simulink model "w3_warplab_agc"  (Simulink 7.7)
settings: Solver=ode45  StartTime=0.0  StopTime=1e4  RelTol=1e-3
PostLoadFcn:
  | w3_warplab_agc_init
InitFcn:
  | w3_warplab_agc_init
StartFcn:
  | w3_warplab_agc_init
undefined symbols (not defined in the file): gcbh, PHY_CONFIG_PKT_DET_CORR_THRESH, PHY_CONFIG_PKT_DET_ENERGY_THRESH, PHY_CONFIG_PKT_DET_MIN_DURR, xlBlockLoadCallback, xlGetNormalizedPeriod
libraries: xbsIndex_r4 x1039, xbsEDKLib_r4 x1, simulink x1
(part 2 of 7)

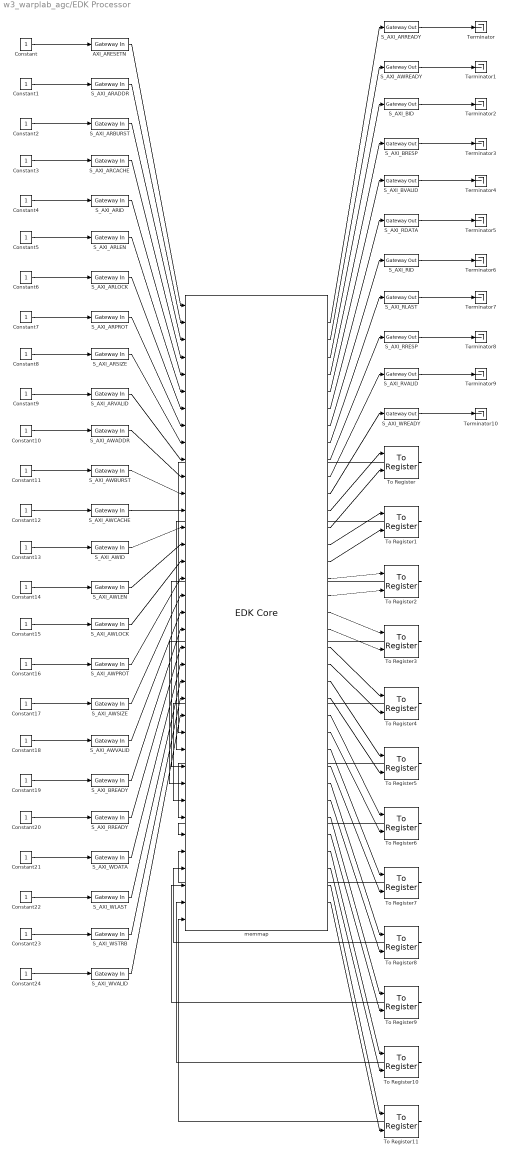
== system w3_warplab_agc/EDK Processor ==
  AXI_ARESETN : xbsIndex_r4/Gateway In  gui_display_data_type=Fixed-point  arith_type=Boolean  n_bits=16  bin_pt=14  preci_type=Single  exp_width=8  frac_width=24  quantization="Round  (unbiased: +/- Inf)"  overflow=Saturate  period=xlGetNormalizedPeriod()  dbl_ovrd=off  timing_constraint=None  locs_specified=off  LOCs={}  UseAsADC=off  ADCChannel='1'  inherit_from_input=off  hdl_port=on  block_type=gatewayin
  Constant{,1..24} (25 alike) : Constant
  S_AXI_ARADDR : xbsIndex_r4/Gateway In  gui_display_data_type=Fixed-point  arith_type=Unsigned  n_bits=32  bin_pt=0  preci_type=Single  exp_width=8  frac_width=24  quantization="Round  (unbiased: +/- Inf)"  overflow=Saturate  period=xlGetNormalizedPeriod()  dbl_ovrd=off  timing_constraint=None  locs_specified=off  LOCs={}  UseAsADC=off  ADCChannel='1'  inherit_from_input=off  hdl_port=on  block_type=gatewayin
  S_AXI_ARBURST : xbsIndex_r4/Gateway In  gui_display_data_type=Fixed-point  arith_type=Unsigned  n_bits=2  bin_pt=0  preci_type=Single  exp_width=8  frac_width=24  quantization="Round  (unbiased: +/- Inf)"  overflow=Saturate  period=xlGetNormalizedPeriod()  dbl_ovrd=off  timing_constraint=None  locs_specified=off  LOCs={}  UseAsADC=off  ADCChannel='1'  inherit_from_input=off  hdl_port=on  block_type=gatewayin
  S_AXI_ARCACHE : xbsIndex_r4/Gateway In  gui_display_data_type=Fixed-point  arith_type=Unsigned  n_bits=4  bin_pt=0  preci_type=Single  exp_width=8  frac_width=24  quantization="Round  (unbiased: +/- Inf)"  overflow=Saturate  period=xlGetNormalizedPeriod()  dbl_ovrd=off  timing_constraint=None  locs_specified=off  LOCs={}  UseAsADC=off  ADCChannel='1'  inherit_from_input=off  hdl_port=on  block_type=gatewayin
  S_AXI_ARID : xbsIndex_r4/Gateway In  gui_display_data_type=Fixed-point  arith_type=Unsigned  n_bits=8  bin_pt=0  preci_type=Single  exp_width=8  frac_width=24  quantization="Round  (unbiased: +/- Inf)"  overflow=Saturate  period=xlGetNormalizedPeriod()  dbl_ovrd=off  timing_constraint=None  locs_specified=off  LOCs={}  UseAsADC=off  ADCChannel='1'  inherit_from_input=off  hdl_port=on  block_type=gatewayin
  S_AXI_ARLEN : xbsIndex_r4/Gateway In  gui_display_data_type=Fixed-point  arith_type=Unsigned  n_bits=8  bin_pt=0  preci_type=Single  exp_width=8  frac_width=24  quantization="Round  (unbiased: +/- Inf)"  overflow=Saturate  period=xlGetNormalizedPeriod()  dbl_ovrd=off  timing_constraint=None  locs_specified=off  LOCs={}  UseAsADC=off  ADCChannel='1'  inherit_from_input=off  hdl_port=on  block_type=gatewayin
  S_AXI_ARLOCK : xbsIndex_r4/Gateway In  gui_display_data_type=Fixed-point  arith_type=Unsigned  n_bits=2  bin_pt=0  preci_type=Single  exp_width=8  frac_width=24  quantization="Round  (unbiased: +/- Inf)"  overflow=Saturate  period=xlGetNormalizedPeriod()  dbl_ovrd=off  timing_constraint=None  locs_specified=off  LOCs={}  UseAsADC=off  ADCChannel='1'  inherit_from_input=off  hdl_port=on  block_type=gatewayin
  S_AXI_ARPROT : xbsIndex_r4/Gateway In  gui_display_data_type=Fixed-point  arith_type=Unsigned  n_bits=3  bin_pt=0  preci_type=Single  exp_width=8  frac_width=24  quantization="Round  (unbiased: +/- Inf)"  overflow=Saturate  period=xlGetNormalizedPeriod()  dbl_ovrd=off  timing_constraint=None  locs_specified=off  LOCs={}  UseAsADC=off  ADCChannel='1'  inherit_from_input=off  hdl_port=on  block_type=gatewayin
  S_AXI_ARREADY : xbsIndex_r4/Gateway Out  inherit_from_input=off  hdl_port=on  timing_constraint=None  locs_specified=off  LOCs={}  UseAsDAC=off  DACChannel='1'  block_type=gatewayout
  S_AXI_ARSIZE : xbsIndex_r4/Gateway In  gui_display_data_type=Fixed-point  arith_type=Unsigned  n_bits=3  bin_pt=0  preci_type=Single  exp_width=8  frac_width=24  quantization="Round  (unbiased: +/- Inf)"  overflow=Saturate  period=xlGetNormalizedPeriod()  dbl_ovrd=off  timing_constraint=None  locs_specified=off  LOCs={}  UseAsADC=off  ADCChannel='1'  inherit_from_input=off  hdl_port=on  block_type=gatewayin
  S_AXI_ARVALID : xbsIndex_r4/Gateway In  gui_display_data_type=Fixed-point  arith_type=Boolean  n_bits=16  bin_pt=14  preci_type=Single  exp_width=8  frac_width=24  quantization="Round  (unbiased: +/- Inf)"  overflow=Saturate  period=xlGetNormalizedPeriod()  dbl_ovrd=off  timing_constraint=None  locs_specified=off  LOCs={}  UseAsADC=off  ADCChannel='1'  inherit_from_input=off  hdl_port=on  block_type=gatewayin
  S_AXI_AWADDR : xbsIndex_r4/Gateway In  gui_display_data_type=Fixed-point  arith_type=Unsigned  n_bits=32  bin_pt=0  preci_type=Single  exp_width=8  frac_width=24  quantization="Round  (unbiased: +/- Inf)"  overflow=Saturate  period=xlGetNormalizedPeriod()  dbl_ovrd=off  timing_constraint=None  locs_specified=off  LOCs={}  UseAsADC=off  ADCChannel='1'  inherit_from_input=off  hdl_port=on  block_type=gatewayin
  S_AXI_AWBURST : xbsIndex_r4/Gateway In  gui_display_data_type=Fixed-point  arith_type=Unsigned  n_bits=2  bin_pt=0  preci_type=Single  exp_width=8  frac_width=24  quantization="Round  (unbiased: +/- Inf)"  overflow=Saturate  period=xlGetNormalizedPeriod()  dbl_ovrd=off  timing_constraint=None  locs_specified=off  LOCs={}  UseAsADC=off  ADCChannel='1'  inherit_from_input=off  hdl_port=on  block_type=gatewayin
  S_AXI_AWCACHE : xbsIndex_r4/Gateway In  gui_display_data_type=Fixed-point  arith_type=Unsigned  n_bits=4  bin_pt=0  preci_type=Single  exp_width=8  frac_width=24  quantization="Round  (unbiased: +/- Inf)"  overflow=Saturate  period=xlGetNormalizedPeriod()  dbl_ovrd=off  timing_constraint=None  locs_specified=off  LOCs={}  UseAsADC=off  ADCChannel='1'  inherit_from_input=off  hdl_port=on  block_type=gatewayin
  S_AXI_AWID : xbsIndex_r4/Gateway In  gui_display_data_type=Fixed-point  arith_type=Unsigned  n_bits=8  bin_pt=0  preci_type=Single  exp_width=8  frac_width=24  quantization="Round  (unbiased: +/- Inf)"  overflow=Saturate  period=xlGetNormalizedPeriod()  dbl_ovrd=off  timing_constraint=None  locs_specified=off  LOCs={}  UseAsADC=off  ADCChannel='1'  inherit_from_input=off  hdl_port=on  block_type=gatewayin
  S_AXI_AWLEN : xbsIndex_r4/Gateway In  gui_display_data_type=Fixed-point  arith_type=Unsigned  n_bits=8  bin_pt=0  preci_type=Single  exp_width=8  frac_width=24  quantization="Round  (unbiased: +/- Inf)"  overflow=Saturate  period=xlGetNormalizedPeriod()  dbl_ovrd=off  timing_constraint=None  locs_specified=off  LOCs={}  UseAsADC=off  ADCChannel='1'  inherit_from_input=off  hdl_port=on  block_type=gatewayin
  S_AXI_AWLOCK : xbsIndex_r4/Gateway In  gui_display_data_type=Fixed-point  arith_type=Unsigned  n_bits=2  bin_pt=0  preci_type=Single  exp_width=8  frac_width=24  quantization="Round  (unbiased: +/- Inf)"  overflow=Saturate  period=xlGetNormalizedPeriod()  dbl_ovrd=off  timing_constraint=None  locs_specified=off  LOCs={}  UseAsADC=off  ADCChannel='1'  inherit_from_input=off  hdl_port=on  block_type=gatewayin
  S_AXI_AWPROT : xbsIndex_r4/Gateway In  gui_display_data_type=Fixed-point  arith_type=Unsigned  n_bits=3  bin_pt=0  preci_type=Single  exp_width=8  frac_width=24  quantization="Round  (unbiased: +/- Inf)"  overflow=Saturate  period=xlGetNormalizedPeriod()  dbl_ovrd=off  timing_constraint=None  locs_specified=off  LOCs={}  UseAsADC=off  ADCChannel='1'  inherit_from_input=off  hdl_port=on  block_type=gatewayin
  S_AXI_AWREADY : xbsIndex_r4/Gateway Out  inherit_from_input=off  hdl_port=on  timing_constraint=None  locs_specified=off  LOCs={}  UseAsDAC=off  DACChannel='1'  block_type=gatewayout
  S_AXI_AWSIZE : xbsIndex_r4/Gateway In  gui_display_data_type=Fixed-point  arith_type=Unsigned  n_bits=3  bin_pt=0  preci_type=Single  exp_width=8  frac_width=24  quantization="Round  (unbiased: +/- Inf)"  overflow=Saturate  period=xlGetNormalizedPeriod()  dbl_ovrd=off  timing_constraint=None  locs_specified=off  LOCs={}  UseAsADC=off  ADCChannel='1'  inherit_from_input=off  hdl_port=on  block_type=gatewayin
  S_AXI_AWVALID : xbsIndex_r4/Gateway In  gui_display_data_type=Fixed-point  arith_type=Boolean  n_bits=16  bin_pt=14  preci_type=Single  exp_width=8  frac_width=24  quantization="Round  (unbiased: +/- Inf)"  overflow=Saturate  period=xlGetNormalizedPeriod()  dbl_ovrd=off  timing_constraint=None  locs_specified=off  LOCs={}  UseAsADC=off  ADCChannel='1'  inherit_from_input=off  hdl_port=on  block_type=gatewayin
  S_AXI_BID : xbsIndex_r4/Gateway Out  inherit_from_input=off  hdl_port=on  timing_constraint=None  locs_specified=off  LOCs={}  UseAsDAC=off  DACChannel='1'  block_type=gatewayout
  S_AXI_BREADY : xbsIndex_r4/Gateway In  gui_display_data_type=Fixed-point  arith_type=Boolean  n_bits=16  bin_pt=14  preci_type=Single  exp_width=8  frac_width=24  quantization="Round  (unbiased: +/- Inf)"  overflow=Saturate  period=xlGetNormalizedPeriod()  dbl_ovrd=off  timing_constraint=None  locs_specified=off  LOCs={}  UseAsADC=off  ADCChannel='1'  inherit_from_input=off  hdl_port=on  block_type=gatewayin
  S_AXI_BRESP : xbsIndex_r4/Gateway Out  inherit_from_input=off  hdl_port=on  timing_constraint=None  locs_specified=off  LOCs={}  UseAsDAC=off  DACChannel='1'  block_type=gatewayout
  S_AXI_BVALID : xbsIndex_r4/Gateway Out  inherit_from_input=off  hdl_port=on  timing_constraint=None  locs_specified=off  LOCs={}  UseAsDAC=off  DACChannel='1'  block_type=gatewayout
  S_AXI_RDATA : xbsIndex_r4/Gateway Out  inherit_from_input=off  hdl_port=on  timing_constraint=None  locs_specified=off  LOCs={}  UseAsDAC=off  DACChannel='1'  block_type=gatewayout
  S_AXI_RID : xbsIndex_r4/Gateway Out  inherit_from_input=off  hdl_port=on  timing_constraint=None  locs_specified=off  LOCs={}  UseAsDAC=off  DACChannel='1'  block_type=gatewayout
  S_AXI_RLAST : xbsIndex_r4/Gateway Out  inherit_from_input=off  hdl_port=on  timing_constraint=None  locs_specified=off  LOCs={}  UseAsDAC=off  DACChannel='1'  block_type=gatewayout
  S_AXI_RREADY : xbsIndex_r4/Gateway In  gui_display_data_type=Fixed-point  arith_type=Boolean  n_bits=16  bin_pt=14  preci_type=Single  exp_width=8  frac_width=24  quantization="Round  (unbiased: +/- Inf)"  overflow=Saturate  period=xlGetNormalizedPeriod()  dbl_ovrd=off  timing_constraint=None  locs_specified=off  LOCs={}  UseAsADC=off  ADCChannel='1'  inherit_from_input=off  hdl_port=on  block_type=gatewayin
  S_AXI_RRESP : xbsIndex_r4/Gateway Out  inherit_from_input=off  hdl_port=on  timing_constraint=None  locs_specified=off  LOCs={}  UseAsDAC=off  DACChannel='1'  block_type=gatewayout
  S_AXI_RVALID : xbsIndex_r4/Gateway Out  inherit_from_input=off  hdl_port=on  timing_constraint=None  locs_specified=off  LOCs={}  UseAsDAC=off  DACChannel='1'  block_type=gatewayout
  S_AXI_WDATA : xbsIndex_r4/Gateway In  gui_display_data_type=Fixed-point  arith_type=Unsigned  n_bits=32  bin_pt=0  preci_type=Single  exp_width=8  frac_width=24  quantization="Round  (unbiased: +/- Inf)"  overflow=Saturate  period=xlGetNormalizedPeriod()  dbl_ovrd=off  timing_constraint=None  locs_specified=off  LOCs={}  UseAsADC=off  ADCChannel='1'  inherit_from_input=off  hdl_port=on  block_type=gatewayin
  S_AXI_WLAST : xbsIndex_r4/Gateway In  gui_display_data_type=Fixed-point  arith_type=Boolean  n_bits=16  bin_pt=14  preci_type=Single  exp_width=8  frac_width=24  quantization="Round  (unbiased: +/- Inf)"  overflow=Saturate  period=xlGetNormalizedPeriod()  dbl_ovrd=off  timing_constraint=None  locs_specified=off  LOCs={}  UseAsADC=off  ADCChannel='1'  inherit_from_input=off  hdl_port=on  block_type=gatewayin
  S_AXI_WREADY : xbsIndex_r4/Gateway Out  inherit_from_input=off  hdl_port=on  timing_constraint=None  locs_specified=off  LOCs={}  UseAsDAC=off  DACChannel='1'  block_type=gatewayout
  S_AXI_WSTRB : xbsIndex_r4/Gateway In  gui_display_data_type=Fixed-point  arith_type=Unsigned  n_bits=4  bin_pt=0  preci_type=Single  exp_width=8  frac_width=24  quantization="Round  (unbiased: +/- Inf)"  overflow=Saturate  period=xlGetNormalizedPeriod()  dbl_ovrd=off  timing_constraint=None  locs_specified=off  LOCs={}  UseAsADC=off  ADCChannel='1'  inherit_from_input=off  hdl_port=on  block_type=gatewayin
  S_AXI_WVALID : xbsIndex_r4/Gateway In  gui_display_data_type=Fixed-point  arith_type=Boolean  n_bits=16  bin_pt=14  preci_type=Single  exp_width=8  frac_width=24  quantization="Round  (unbiased: +/- Inf)"  overflow=Saturate  period=xlGetNormalizedPeriod()  dbl_ovrd=off  timing_constraint=None  locs_specified=off  LOCs={}  UseAsADC=off  ADCChannel='1'  inherit_from_input=off  hdl_port=on  block_type=gatewayin
  Terminator{,1..10} (11 alike) : Terminator
  To Register : xbsIndex_r4/To Register  shared_memory_name='TIMING_RESET'  init=0  ownership=Owned and initialized elsewhere  explicit_data_type=on  gui_display_data_type=Fixed-point  arith_type=Unsigned  n_bits=32  bin_pt=0  preci_type=Single  dbl_ovrd=off  block_type=toreg
      settings: AttributesFormatString=<< %<shared_memory_name> >>  infoedit="Register block that writes data to a shared memory register.  Delay of one sample period."
  To Register1 : xbsIndex_r4/To Register  shared_memory_name='RSSI_PWR_CALIB'  init=0  ownership=Owned and initialized elsewhere  explicit_data_type=on  gui_display_data_type=Fixed-point  arith_type=Unsigned  n_bits=32  bin_pt=0  preci_type=Single  dbl_ovrd=off  block_type=toreg
      settings: AttributesFormatString=<< %<shared_memory_name> >>  infoedit="Register block that writes data to a shared memory register.  Delay of one sample period."
  To Register10 : xbsIndex_r4/To Register  shared_memory_name='RX_LENGTH'  init=0  ownership=Owned and initialized elsewhere  explicit_data_type=on  gui_display_data_type=Fixed-point  arith_type=Unsigned  n_bits=32  bin_pt=0  preci_type=Single  dbl_ovrd=off  block_type=toreg
      settings: AttributesFormatString=<< %<shared_memory_name> >>  infoedit="Register block that writes data to a shared memory register.  Delay of one sample period."
  To Register11 : xbsIndex_r4/To Register  shared_memory_name='TIMING_DCO'  init=0  ownership=Owned and initialized elsewhere  explicit_data_type=on  gui_display_data_type=Fixed-point  arith_type=Unsigned  n_bits=32  bin_pt=0  preci_type=Single  dbl_ovrd=off  block_type=toreg
      settings: AttributesFormatString=<< %<shared_memory_name> >>  infoedit="Register block that writes data to a shared memory register.  Delay of one sample period."
  To Register2 : xbsIndex_r4/To Register  shared_memory_name='IIR_COEF_B0'  init=0  ownership=Owned and initialized elsewhere  explicit_data_type=on  gui_display_data_type=Fixed-point  arith_type=Unsigned  n_bits=18  bin_pt=17  preci_type=Single  dbl_ovrd=off  block_type=toreg
      settings: AttributesFormatString=<< %<shared_memory_name> >>  infoedit="Register block that writes data to a shared memory register.  Delay of one sample period."
  To Register3 : xbsIndex_r4/To Register  shared_memory_name='IIR_COEF_A1'  init=0  ownership=Owned and initialized elsewhere  explicit_data_type=on  gui_display_data_type=Fixed-point  arith_type="Signed  (2's comp)"  n_bits=18  bin_pt=17  preci_type=Single  dbl_ovrd=off  block_type=toreg
      settings: AttributesFormatString=<< %<shared_memory_name> >>  infoedit="Register block that writes data to a shared memory register.  Delay of one sample period."
  To Register4 : xbsIndex_r4/To Register  shared_memory_name='RESET'  init=0  ownership=Owned and initialized elsewhere  explicit_data_type=on  gui_display_data_type=Fixed-point  arith_type=Unsigned  n_bits=32  bin_pt=0  preci_type=Single  dbl_ovrd=off  block_type=toreg
      settings: AttributesFormatString=<< %<shared_memory_name> >>  infoedit="Register block that writes data to a shared memory register.  Delay of one sample period."
  To Register5 : xbsIndex_r4/To Register  shared_memory_name='TIMING_AGC'  init=0  ownership=Owned and initialized elsewhere  explicit_data_type=on  gui_display_data_type=Fixed-point  arith_type=Unsigned  n_bits=32  bin_pt=0  preci_type=Single  dbl_ovrd=off  block_type=toreg
      settings: AttributesFormatString=<< %<shared_memory_name> >>  infoedit="Register block that writes data to a shared memory register.  Delay of one sample period."
  To Register6 : xbsIndex_r4/To Register  shared_memory_name='TARGET'  init=0  ownership=Owned and initialized elsewhere  explicit_data_type=on  gui_display_data_type=Fixed-point  arith_type=Unsigned  n_bits=32  bin_pt=0  preci_type=Single  dbl_ovrd=off  block_type=toreg
      settings: AttributesFormatString=<< %<shared_memory_name> >>  infoedit="Register block that writes data to a shared memory register.  Delay of one sample period."
  To Register7 : xbsIndex_r4/To Register  shared_memory_name='CONFIG'  init=0  ownership=Owned and initialized elsewhere  explicit_data_type=on  gui_display_data_type=Fixed-point  arith_type=Unsigned  n_bits=32  bin_pt=0  preci_type=Single  dbl_ovrd=off  block_type=toreg
      settings: AttributesFormatString=<< %<shared_memory_name> >>  infoedit="Register block that writes data to a shared memory register.  Delay of one sample period."
  To Register8 : xbsIndex_r4/To Register  shared_memory_name='RESET_MODE'  init=0  ownership=Owned and initialized elsewhere  explicit_data_type=on  gui_display_data_type=Fixed-point  arith_type=Unsigned  n_bits=32  bin_pt=0  preci_type=Single  dbl_ovrd=off  block_type=toreg
      settings: AttributesFormatString=<< %<shared_memory_name> >>  infoedit="Register block that writes data to a shared memory register.  Delay of one sample period."
  To Register9 : xbsIndex_r4/To Register  shared_memory_name='AGC_OVERRIDE'  init=0  ownership=Owned and initialized elsewhere  explicit_data_type=on  gui_display_data_type=Fixed-point  arith_type=Unsigned  n_bits=32  bin_pt=0  preci_type=Single  dbl_ovrd=off  block_type=toreg
      settings: AttributesFormatString=<< %<shared_memory_name> >>  infoedit="Register block that writes data to a shared memory register.  Delay of one sample period."
  memmap : xbsEDKLib_r4/EDK Core  sim_method=Inactive  xmp=xmp  blockname=blockname  dual_clock=dual_clock  procinfo=procinfo  bus_type=bus_type  memxtable=memxtable  memmap_hdlcontent=|  config={'inports'=>[{'arith_type'=>2.00000000000000000,'bin_pt'=>0.00000000000000000,'name'=>'AXI_ARESETN','width'=>0},{'arith_type'=>2.00000000000000000,'bin_pt'=>0.00000000000000000,'name'=>'S_AXI_ARADDR','width'=>32},{'arith_type'=>2.00000000000000000,'bin_pt'=>0.00000000000000000,'name'=>'S_AXI_ARBURST','width'=>2},{'arith_type'=>2.00000000000000000,'bin_pt'=>0.00000000000000000,'name'=>'S_AXI_ARCACHE','width'=>4},{'arith_type'=>2.00000000000000000,'bin_pt'=>0.00000000000000000,'name'=>'S_AXI_ARID','width'=>8},{'arith_type'=>2.00000000000000000,'bin_pt'=>0.00000000000000000,'name'=>'S_AXI_ARLEN','width'=>8},{'arith_type'=>2.00000000000000000,'bin_pt'=>0.00000000000000000,'name'=>'S_AXI_ARLOCK','width'=>2},{'arith_type'=>2.00000000000000000,'bin_pt'=>0.00000000000000000,'name'=>'S_AXI_ARPROT','width'=>3},{'arith_type'=>2.00000000000000000,'bin_pt'=>0.00000000000000000,'name'=>'S_AXI_ARSIZE','width'=>3},{'arith_type'=>2.00000000000000000,'bin_pt'=>0.00000000000000000,'name'=>'S_AXI_ARVALID','width'=>0},{'arith_type'=>2.00000000000000000,'bin_pt'=>0.00000000000000000,'name'=>'S_AXI_AWADDR','width'=>32},{'arith_type'=>2.00000000000000000,'bin_pt'=>0.00000000000000000,'name'=>'S_AXI_AWBURST','width'=>2},{'arith_type'=>2.00000000000000000,'bin_pt'=>0.00000000000000000,'name'=>'S_AXI_AWCACHE','width'=>4},{'arith_type'=>2.00000000000000000,'bin_pt'=>0.00000000000000000,'name'=>'S_AXI_AWID','width'=>8},{'arith_type'=>2.00000000000000000,'bin_pt'=>0.00000000000000000,'name'=>'S_AXI_AWLEN','width'=>8},{'arith_type'=>2.00000000000000000,'bin_pt'=>0.00000000000000000,'name'=>'S_AXI_AWLOCK','width'=>2},{'arith_type'=>2.00000000000000000,'bin_pt'=>0.00000000000000000,'name'=>'S_AXI_AWPROT','width'=>3},{'arith_type'=>2.00000000000000000,'bin_pt'=>0.00000000000000000,'name'=>'S_AXI_AWSIZE','width'=>3},{'arith_type'=>2.00000000000000000,'bin_pt'=>0.00000000000000000,'name'=>'S_AXI_AWVALID','width'=>0},{'arith_type'=>2.00000000000000000,'bin_pt'=>0.00000000000000000,'name'=>'S_AXI_BREADY','width'=>0},{'arith_type'=>2.00000000000000000,'bin_pt'=>0.00000000000000000,'name'=>'S_AXI_RREADY','width'=>0},{'arith_type'=>2.00000000000000000,'bin_pt'=>0.00000000000000000,'name'=>'S_AXI_WDATA','width'=>32},{'arith_type'=>2.00000000000000000,'bin_pt'=>0.00000000000000000,'name'=>'S_AXI_WLAST','width'=>0},{'arith_type'=>2.00000000000000000,'bin_pt'=>0.00000000000000000,'name'=>'S_AXI_WSTRB','width'=>4},{'arith_type'=>2.00000000000000000,'bin_pt'=>0.00000000000000000,'name'=>'S_AXI_WVALID','width'=>0},{'arith_type'=>2,'bin_pt'=>0,'name'=>'sm_TIMING_RESET_dout','width'=>32},{'arith_type'=>2,'bin_pt'=>0,'name'=>'sm_RSSI_PWR_CALIB_dout','width'=>32},{'arith_type'=>2,'bin_pt'=>17,'name'=>'sm_IIR_COEF_B0_dout','width'=>18},{'arith_type'=>1,'bin_pt'=>17,'name'=>'sm_IIR_COEF_A1_dout','width'=>18},{'arith_type'=>2,'bin_pt'=>0,'name'=>'sm_RESET_dout','width'=>32},{'arith_type'=>2,'bin_pt'=>0,'name'=>'sm_TIMING_AGC_dout','width'=>32},{'arith_type'=>2,'bin_pt'=>0,'name'=>'sm_TARGET_dout','width'=>32},{'arith_type'=>2,'bin_pt'=>0,'name'=>'sm_CONFIG_dout','width'=>32},{'arith_type'=>2,'bin_pt'=>0,'name'=>'sm_RESET_MODE_dout','width'=>32},{'arith_type'=>2,'bin_pt'=>0,'name'=>'sm_AGC_OVERRIDE_dout','width'=>32},{'arith_type'=>2,'bin_pt'=>0,'name'=>'sm_RX_LENGTH_dout','width'=>32},{'arith_type'=>2,'bin_pt'=>0,'name'=>'sm_TIMING_DCO_dout','width'=>32}],'outports'=>[{'arith_type'=>2.00000000000000000,'bin_pt'=>0.00000000000000000,'name'=>'S_AXI_ARREADY','width'=>0},{'arith_type'=>2.00000000000000000,'bin_pt'=>0.00000000000000000,'name'=>'S_AXI_AWREADY','width'=>0},{'arith_type'=>2.00000000000000000,'bin_pt'=>0.00000000000000000,'name'=>'S_AXI_BID','width'=>8},{'arith_type'=>2.00000000000000000,'bin_pt'=>0.00000000000000000,'name'=>'S_AXI_BRESP','width'=>2},{'arith_type'=>2.00000000000000000,'bin_pt'=>0.00000000000000000,'name'=>'S_AXI_BVALID','width'=>0},{'arith_type'=>2.00000000000000000,'bin_pt'=>0.00000000000000000,'name'=>'S_AXI_RDATA','width'=>32},{'arith_type'=>2.00000000000000000,'bin_pt'=>0.00000000000000000,'name'=>'S_AXI_RID','width'=>8},{'arith_type'=>2.00000000000000000,'bin_pt'=>0.00000000000000000,'name'=>'S_AXI_RLAST','width'=>0},{'arith_type'=>2.00000000000000000,'bin_pt'=>0.00000000000000000,'name'=>'S_AXI_RRESP','width'=>2},{'arith_type'=>2.00000000000000000,'bin_pt'=>0.00000000000000000,'name'=>'S_AXI_RVALID','width'=>0},{'arith_type'=>2.00000000000000000,'bin_pt'=>0.00000000000000000,'name'=>'S_AXI_WREADY','width'=>0},{'arith_type'=>2,'bin_pt'=>0,'name'=>'sm_TIMING_RESET_din','width'=>32},{'arith_type'=>2.00000000000000000,'bin_pt'=>0.00000000000000000,'name'=>'sm_TIMING_RESET_en','width'=>0.00000000000000000},{'arith_type'=>2,'bin_pt'=>0,'name'=>'sm_RSSI_PWR_CALIB_din','width'=>32},{'arith_type'=>2.00000000000000000,'bin_pt'=>0.00000000000000000,'name'=>'sm_RSSI_PWR_CALIB_en','width'=>0.00000000000000000},{'arith_type'=>2,'bin_pt'=>17,'name'=>'sm_IIR_COEF_B0_din','width'=>18},{'arith_type'=>2.00000000000000000,'bin_pt'=>0.00000000000000000,'name'=>'sm_IIR_COEF_B0_en','width'=>0.00000000000000000},{'arith_type'=>1,'bin_pt'=>17,'name'=>'sm_IIR_COEF_A1_din','width'=>18},{'arith_type'=>2.00000000000000000,'bin_pt'=>0.00000000000000000,'name'=>'sm_IIR_COEF_A1_en','width'=>0.00000000000000000},{'arith_type'=>2,'bin_pt'=>0,'name'=>'sm_RESET_din','width'=>32},{'arith_type'=>2.00000000000000000,'bin_pt'=>0.00000000000000000,'name'=>'sm_RESET_en','width'=>0.00000000000000000},{'arith_type'=>2,'bin_pt'=>0,'name'=>'sm_TIMING_AGC_din','width'=>32},{'arith_type'=>2.00000000000000000,'bin_pt'=>0.00000000000000000,'name'=>'sm_TIMING_AGC_en','width'=>0.00000000000000000},{'arith_type'=>2,'bin_pt'=>0,'name'=>'sm_TARGET_din','width'=>32},{'arith_type'=>2.00000000000000000,'bin_pt'=>0.00000000000000000,'name'=>'sm_TARGET_en','width'=>0.00000000000000000},{'arith_type'=>2,'bin_pt'=>0,'name'=>'sm_CONFIG_din','width'=>32},{'arith_type'=>2.00000000000000000,'bin_pt'=>0.00000000000000000,'name'=>'sm_CONFIG_en','width'=>0.00000000000000000},{'arith_type'=>2,'bin_pt'=>0,'name'=>'sm_RESET_MODE_din','width'=>32},{'arith_type'=>2.00000000000000000,'bin_pt'=>0.00000000000000000,'name'=>'sm_RESET_MODE_en','width'=>0.00000000000000000},{'arith_type'=>2,'bin_pt'=>0,'name'=>'sm_AGC_OVERRIDE_din','width'=>32},{'arith_type'=>2.00000000000000000,'bin_pt'=>0.00000000000000000,'name'=>'sm_AGC_OVERRIDE_en','width'=>0.00000000000000000},{'arith_type'=>2,'bin_pt'=>0,'name'=>'sm_RX_LENGTH_din','width'=>32},{'arith_type'=>2.00000000000000000,'bin_pt'=>0.00000000000000000,'name'=>'sm_RX_LENGTH_en','width'=>0.00000000000000000},{'arith_type'=>2,'bin_pt'=>0,'name'=>'sm_TIMING_DCO_din','width'=>32},{'arith_type'=>2.00000000000000000,'bin_pt'=>0.00000000000000000,'name'=>'sm_TIMING_DCO_en','width'=>0.00000000000000000}]}  inheritDeviceType=inheritDeviceType  block_type=edkcore
      | library IEEE;
      | use IEEE.std_logic_1164.all;
      | use IEEE.numeric_std.all;
      | 
      | entity axi_sgiface is
      |     generic (
      |         -- AXI specific.
      |         -- TODO: need to figure out a way to pass these generics from outside
      |         C_S_AXI_SUPPORT_BURST   : integer := 0;
      |         -- TODO: fix the internal ID width to 8
      |         C_S_AXI_ID_WIDTH        : integer := 8;
      |         C_S_AXI_DATA_WIDTH      : integer := 32;
      |         C_S_AXI_ADDR_WIDTH      : integer := 32;
      |         C_S_AXI_TOTAL_ADDR_LEN  : integer := 12;
      |         C_S_AXI_LINEAR_ADDR_LEN : integer := 8;
      |         C_S_AXI_BANK_ADDR_LEN   : integer := 2;
      |         C_S_AXI_AWLEN_WIDTH     : integer := 8;
      |         C_S_AXI_ARLEN_WIDTH     : integer := 8
      |     );
      |     port (
      |         -- General.
      |         AXI_AClk      : in  std_logic;
      |         AXI_AResetN    : in  std_logic;
      |         -- not used
      |         AXI_Ce        : in  std_logic;
      |   
      |         -- AXI Port.
      |         S_AXI_AWADDR  : in  std_logic_vector(C_S_AXI_ADDR_WIDTH-1 downto 0);
      |         S_AXI_AWID    : in  std_logic_vector(C_S_AXI_ID_WIDTH-1 downto 0);
      |         S_AXI_AWLEN   : in  std_logic_vector(C_S_AXI_AWLEN_WIDTH-1 downto 0);
      |         S_AXI_AWSIZE  : in  std_logic_vector(2 downto 0);
      |         S_AXI_AWBURST : in  std_logic_vector(1 downto 0);
      |         S_AXI_AWLOCK  : in  std_logic_vector(1 downto 0);
      |         S_AXI_AWCACHE : in  std_logic_vector(3 downto 0);
      |         S_AXI_AWPROT  : in  std_logic_vector(2 downto 0);
      |         S_AXI_AWVALID : in  std_logic;
      |         S_AXI_AWREADY : out std_logic;
      |         
      |         S_AXI_WLAST   : in  std_logic;
      |         S_AXI_WDATA   : in  std_logic_vector(C_S_AXI_DATA_WIDTH-1 downto 0);
      |         S_AXI_WSTRB   : in  std_logic_vector((C_S_AXI_DATA_WIDTH/8)-1 downto 0);
      |         S_AXI_WVALID  : in  std_logic;
      |         S_AXI_WREADY  : out std_logic;
      |         
      |         S_AXI_BRESP   : out std_logic_vector(1 downto 0);
      |         S_AXI_BID     : out std_logic_vector(C_S_AXI_ID_WIDTH-1 downto 0);
      |         S_AXI_BVALID  : out std_logic;
      |         S_AXI_BREADY  : in  std_logic;
      |         
      |         S_AXI_ARADDR  : in  std_logic_vector(C_S_AXI_ADDR_WIDTH-1 downto 0);
      |         S_AXI_ARID    : in  std_logic_vector(C_S_AXI_ID_WIDTH-1 downto 0);
      |         S_AXI_ARLEN   : in  std_logic_vector(C_S_AXI_ARLEN_WIDTH-1 downto 0);
      |         S_AXI_ARSIZE  : in  std_logic_vector(2 downto 0);
      |         S_AXI_ARBURST : in  std_logic_vector(1 downto 0);
      |         S_AXI_ARLOCK  : in  std_logic_vector(1 downto 0);
      |         S_AXI_ARCACHE : in  std_logic_vector(3 downto 0);
      |         S_AXI_ARPROT  : in  std_logic_vector(2 downto 0);
      |         S_AXI_ARVALID : in  std_logic;
      |         S_AXI_ARREADY : out std_logic;
      |         
      |         -- 'From Register'
      |         -- 'To Register'
      |         -- 'TIMING_RESET'
      |         sm_TIMING_RESET_dout : in std_logic_vector(32-1 downto 0);
      |         sm_TIMING_RESET_din  : out std_logic_vector(32-1 downto 0);
      |         sm_TIMING_RESET_en   : out std_logic;
      |         -- 'RSSI_PWR_CALIB'
      |         sm_RSSI_PWR_CALIB_dout : in std_logic_vector(32-1 downto 0);
      |         sm_RSSI_PWR_CALIB_din  : out std_logic_vector(32-1 downto 0);
      |         sm_RSSI_PWR_CALIB_en   : out std_logic;
      |         -- 'IIR_COEF_B0'
      |         sm_IIR_COEF_B0_dout : in std_logic_vector(18-1 downto 0);
      |         sm_IIR_COEF_B0_din  : out std_logic_vector(18-1 downto 0);
      |         sm_IIR_COEF_B0_en   : out std_logic;
      |         -- 'IIR_COEF_A1'
      |         sm_IIR_COEF_A1_dout : in std_logic_vector(18-1 downto 0);
      |         sm_IIR_COEF_A1_din  : out std_logic_vector(18-1 downto 0);
      |         sm_IIR_COEF_A1_en   : out std_logic;
      |         -- 'RESET'
      |         sm_RESET_dout : in std_logic_vector(32-1 downto 0);
      |         sm_RESET_din  : out std_logic_vector(32-1 downto 0);
      |         sm_RESET_en   : out std_logic;
      |         -- 'TIMING_AGC'
      |         sm_TIMING_AGC_dout : in std_logic_vector(32-1 downto 0);
      |         sm_TIMING_AGC_din  : out std_logic_vector(32-1 downto 0);
      |         sm_TIMING_AGC_en   : out std_logic;
      |         -- 'TARGET'
      |         sm_TARGET_dout : in std_logic_vector(32-1 downto 0);
      |         sm_TARGET_din  : out std_logic_vector(32-1 downto 0);
      |         sm_TARGET_en   : out std_logic;
      |         -- 'CONFIG'
      |         sm_CONFIG_dout : in std_logic_vector(32-1 downto 0);
      |         sm_CONFIG_din  : out std_logic_vector(32-1 downto 0);
      |         sm_CONFIG_en   : out std_logic;
      |         -- 'RESET_MODE'
      |         sm_RESET_MODE_dout : in std_logic_vector(32-1 downto 0);
      |         sm_RESET_MODE_din  : out std_logic_vector(32-1 downto 0);
      |         sm_RESET_MODE_en   : out std_logic;
      |         -- 'AGC_OVERRIDE'
      |         sm_AGC_OVERRIDE_dout : in std_logic_vector(32-1 downto 0);
      |         sm_AGC_OVERRIDE_din  : out std_logic_vector(32-1 downto 0);
      |         sm_AGC_OVERRIDE_en   : out std_logic;
      |         -- 'RX_LENGTH'
      |         sm_RX_LENGTH_dout : in std_logic_vector(32-1 downto 0);
      |         sm_RX_LENGTH_din  : out std_logic_vector(32-1 downto 0);
      |         sm_RX_LENGTH_en   : out std_logic;
      |         -- 'TIMING_DCO'
      |         sm_TIMING_DCO_dout : in std_logic_vector(32-1 downto 0);
      |         sm_TIMING_DCO_din  : out std_logic_vector(32-1 downto 0);
      |         sm_TIMING_DCO_en   : out std_logic;
      |         -- 'From FIFO'
      |         -- 'To FIFO'
      |         -- 'Shared Memory'
      | 
      |         S_AXI_RLAST   : out std_logic;
      |         S_AXI_RID     : out std_logic_vector(C_S_AXI_ID_WIDTH-1 downto 0);
      |         S_AXI_RDATA   : out std_logic_vector(C_S_AXI_DATA_WIDTH-1 downto 0);
      |         S_AXI_RRESP   : out std_logic_vector(1 downto 0);
      |         S_AXI_RVALID  : out std_logic;
      |         S_AXI_RREADY  : in  std_logic
      |     );
      | end entity axi_sgiface;
      | 
      | architecture IMP of axi_sgiface is
      | 
      | -- Internal signals for write channel.
      | signal S_AXI_BVALID_i       : std_logic;
      | signal S_AXI_BID_i          : std_logic_vector(C_S_AXI_ID_WIDTH-1 downto 0);
      | signal S_AXI_WREADY_i       : std_logic;
      |   
      | -- Internal signals for read channels.
      | signal S_AXI_ARLEN_i        : std_logic_vector(C_S_AXI_ARLEN_WIDTH-1 downto 0);
      | signal S_AXI_RLAST_i        : std_logic;
      | signal S_AXI_RREADY_i       : std_logic;
      | signal S_AXI_RVALID_i       : std_logic;
      | signal S_AXI_RDATA_i        : std_logic_vector(C_S_AXI_DATA_WIDTH-1 downto 0);
      | signal S_AXI_RID_i          : std_logic_vector(C_S_AXI_ID_WIDTH-1 downto 0);
      | 
      | -- for read channel
      | signal read_bank_addr_i     : std_logic_vector(C_S_AXI_BANK_ADDR_LEN-1 downto 0);
      | signal read_linear_addr_i   : std_logic_vector(C_S_AXI_LINEAR_ADDR_LEN-1 downto 0);
      | -- for write channel
      | signal write_bank_addr_i    : std_logic_vector(C_S_AXI_BANK_ADDR_LEN-1 downto 0);
      | signal write_linear_addr_i  : std_logic_vector(C_S_AXI_LINEAR_ADDR_LEN-1 downto 0);
      | 
      | signal reg_bank_out_i       : std_logic_vector(C_S_AXI_DATA_WIDTH-1 downto 0);
      | signal fifo_bank_out_i      : std_logic_vector(C_S_AXI_DATA_WIDTH-1 downto 0);
      | signal shmem_bank_out_i     : std_logic_vector(C_S_AXI_DATA_WIDTH-1 downto 0);
      |     
      | -- 'From Register'
      | -- 'To Register'
      | -- 'TIMING_RESET'
      | signal sm_TIMING_RESET_din_i   : std_logic_vector(C_S_AXI_DATA_WIDTH-1 downto 0);
      | signal sm_TIMING_RESET_en_i    : std_logic;
      | signal sm_TIMING_RESET_dout_i  : std_logic_vector(C_S_AXI_DATA_WIDTH-1 downto 0);
      | -- 'RSSI_PWR_CALIB'
      | signal sm_RSSI_PWR_CALIB_din_i   : std_logic_vector(C_S_AXI_DATA_WIDTH-1 downto 0);
      | signal sm_RSSI_PWR_CALIB_en_i    : std_logic;
      | signal sm_RSSI_PWR_CALIB_dout_i  : std_logic_vector(C_S_AXI_DATA_WIDTH-1 downto 0);
      | -- 'IIR_COEF_B0'
      | signal sm_IIR_COEF_B0_din_i   : std_logic_vector(C_S_AXI_DATA_WIDTH-1 downto 0);
      | signal sm_IIR_COEF_B0_en_i    : std_logic;
      | signal sm_IIR_COEF_B0_dout_i  : std_logic_vector(C_S_AXI_DATA_WIDTH-1 downto 0);
      | -- 'IIR_COEF_A1'
      | signal sm_IIR_COEF_A1_din_i   : std_logic_vector(C_S_AXI_DATA_WIDTH-1 downto 0);
      | signal sm_IIR_COEF_A1_en_i    : std_logic;
      | signal sm_IIR_COEF_A1_dout_i  : std_logic_vector(C_S_AXI_DATA_WIDTH-1 downto 0);
      | -- 'RESET'
      | signal sm_RESET_din_i   : std_logic_vector(C_S_AXI_DATA_WIDTH-1 downto 0);
      | signal sm_RESET_en_i    : std_logic;
      | signal sm_RESET_dout_i  : std_logic_vector(C_S_AXI_DATA_WIDTH-1 downto 0);
      | -- 'TIMING_AGC'
      | signal sm_TIMING_AGC_din_i   : std_logic_vector(C_S_AXI_DATA_WIDTH-1 downto 0);
      | signal sm_TIMING_AGC_en_i    : std_logic;
      | signal sm_TIMING_AGC_dout_i  : std_logic_vector(C_S_AXI_DATA_WIDTH-1 downto 0);
      | -- 'TARGET'
      | signal sm_TARGET_din_i   : std_logic_vector(C_S_AXI_DATA_WIDTH-1 downto 0);
      | signal sm_TARGET_en_i    : std_logic;
      | signal sm_TARGET_dout_i  : std_logic_vector(C_S_AXI_DATA_WIDTH-1 downto 0);
      | -- 'CONFIG'
      | signal sm_CONFIG_din_i   : std_logic_vector(C_S_AXI_DATA_WIDTH-1 downto 0);
      | signal sm_CONFIG_en_i    : std_logic;
      | signal sm_CONFIG_dout_i  : std_logic_vector(C_S_AXI_DATA_WIDTH-1 downto 0);
      | -- 'RESET_MODE'
      | signal sm_RESET_MODE_din_i   : std_logic_vector(C_S_AXI_DATA_WIDTH-1 downto 0);
      | signal sm_RESET_MODE_en_i    : std_logic;
      | signal sm_RESET_MODE_dout_i  : std_logic_vector(C_S_AXI_DATA_WIDTH-1 downto 0);
      | -- 'AGC_OVERRIDE'
      | signal sm_AGC_OVERRIDE_din_i   : std_logic_vector(C_S_AXI_DATA_WIDTH-1 downto 0);
      | signal sm_AGC_OVERRIDE_en_i    : std_logic;
      | signal sm_AGC_OVERRIDE_dout_i  : std_logic_vector(C_S_AXI_DATA_WIDTH-1 downto 0);
      | -- 'RX_LENGTH'
      | signal sm_RX_LENGTH_din_i   : std_logic_vector(C_S_AXI_DATA_WIDTH-1 downto 0);
      | signal sm_RX_LENGTH_en_i    : std_logic;
      | signal sm_RX_LENGTH_dout_i  : std_logic_vector(C_S_AXI_DATA_WIDTH-1 downto 0);
      | -- 'TIMING_DCO'
      | signal sm_TIMING_DCO_din_i   : std_logic_vector(C_S_AXI_DATA_WIDTH-1 downto 0);
      | signal sm_TIMING_DCO_en_i    : std_logic;
      | signal sm_TIMING_DCO_dout_i  : std_logic_vector(C_S_AXI_DATA_WIDTH-1 downto 0);
      | -- 'From FIFO'
      | -- 'To FIFO'
      | -- 'Shared Memory'
      | 
      | type t_read_state is (IDLE, READ_PREP, READ_DATA);
      | signal read_state : t_read_state;
      | 
      | type t_write_state is (IDLE, WRITE_DATA, WRITE_RESPONSE);
      | signal write_state : t_write_state;
      | 
      | type t_memmap_state is (READ, WRITE);
      | signal memmap_state : t_memmap_state;
      | 
      | constant C_READ_PREP_DELAY : std_logic_vector(1 downto 0) := "11";
      | 
      | signal read_prep_counter : std_logic_vector(1 downto 0);
      | signal read_addr_counter : std_logic_vector(C_S_AXI_ARLEN_WIDTH-1 downto 0);
      | signal read_data_counter : std_logic_vector(C_S_AXI_ARLEN_WIDTH-1 downto 0);
      | 
      | -- enable of shared BRAMs
      | signal s_shram_en : std_logic;
      | 
      | signal write_addr_valid : std_logic;
      | signal write_ready : std_logic;
      | 
      | -- 're' of From/To FIFOs
      | signal s_fifo_re : std_logic;
      | -- 'we' of To FIFOs
      | signal s_fifo_we : std_logic;
      | 
      | begin
      | 
      | -- enable for 'Shared Memory' blocks
      | 
      | -- conversion to match with the data bus width
      | -- 'From Register'
      | -- 'To Register'
      | -- 'TIMING_RESET'
      | sm_TIMING_RESET_din     <= sm_TIMING_RESET_din_i(32-1 downto 0);
      | sm_TIMING_RESET_en      <= sm_TIMING_RESET_en_i;
      | gen_sm_TIMING_RESET_dout_i: if (32 < C_S_AXI_DATA_WIDTH) generate
      |     sm_TIMING_RESET_dout_i(C_S_AXI_DATA_WIDTH-1 downto 32) <= (others => '0');
      | end generate gen_sm_TIMING_RESET_dout_i;
      | sm_TIMING_RESET_dout_i(32-1 downto 0) <= sm_TIMING_RESET_dout;
      | -- 'RSSI_PWR_CALIB'
      | sm_RSSI_PWR_CALIB_din     <= sm_RSSI_PWR_CALIB_din_i(32-1 downto 0);
      | sm_RSSI_PWR_CALIB_en      <= sm_RSSI_PWR_CALIB_en_i;
      | gen_sm_RSSI_PWR_CALIB_dout_i: if (32 < C_S_AXI_DATA_WIDTH) generate
      |     sm_RSSI_PWR_CALIB_dout_i(C_S_AXI_DATA_WIDTH-1 downto 32) <= (others => '0');
      | end generate gen_sm_RSSI_PWR_CALIB_dout_i;
      | sm_RSSI_PWR_CALIB_dout_i(32-1 downto 0) <= sm_RSSI_PWR_CALIB_dout;
      | -- 'IIR_COEF_B0'
      | sm_IIR_COEF_B0_din     <= sm_IIR_COEF_B0_din_i(18-1 downto 0);
      | sm_IIR_COEF_B0_en      <= sm_IIR_COEF_B0_en_i;
      | gen_sm_IIR_COEF_B0_dout_i: if (18 < C_S_AXI_DATA_WIDTH) generate
      |     sm_IIR_COEF_B0_dout_i(C_S_AXI_DATA_WIDTH-1 downto 18) <= (others => '0');
      | end generate gen_sm_IIR_COEF_B0_dout_i;
      | sm_IIR_COEF_B0_dout_i(18-1 downto 0) <= sm_IIR_COEF_B0_dout;
      | -- 'IIR_COEF_A1'
      | sm_IIR_COEF_A1_din     <= sm_IIR_COEF_A1_din_i(18-1 downto 0);
      | sm_IIR_COEF_A1_en      <= sm_IIR_COEF_A1_en_i;
      | gen_sm_IIR_COEF_A1_dout_i: if (18 < C_S_AXI_DATA_WIDTH) generate
      |     sm_IIR_COEF_A1_dout_i(C_S_AXI_DATA_WIDTH-1 downto 18) <= (others => '0');
      | end generate gen_sm_IIR_COEF_A1_dout_i;
      | sm_IIR_COEF_A1_dout_i(18-1 downto 0) <= sm_IIR_COEF_A1_dout;
      | -- 'RESET'
      | sm_RESET_din     <= sm_RESET_din_i(32-1 downto 0);
      | sm_RESET_en      <= sm_RESET_en_i;
      | gen_sm_RESET_dout_i: if (32 < C_S_AXI_DATA_WIDTH) generate
      |     sm_RESET_dout_i(C_S_AXI_DATA_WIDTH-1 downto 32) <= (others => '0');
      | end generate gen_sm_RESET_dout_i;
      | sm_RESET_dout_i(32-1 downto 0) <= sm_RESET_dout;
      | -- 'TIMING_AGC'
      | sm_TIMING_AGC_din     <= sm_TIMING_AGC_din_i(32-1 downto 0);
      | sm_TIMING_AGC_en      <= sm_TIMING_AGC_en_i;
      | gen_sm_TIMING_AGC_dout_i: if (32 < C_S_AXI_DATA_WIDTH) generate
      |     sm_TIMING_AGC_dout_i(C_S_AXI_DATA_WIDTH-1 downto 32) <= (others => '0');
      | end generate gen_sm_TIMING_AGC_dout_i;
      | sm_TIMING_AGC_dout_i(32-1 downto 0) <= sm_TIMING_AGC_dout;
      | -- 'TARGET'
      | sm_TARGET_din     <= sm_TARGET_din_i(32-1 downto 0);
      | sm_TARGET_en      <= sm_TARGET_en_i;
      | gen_sm_TARGET_dout_i: if (32 < C_S_AXI_DATA_WIDTH) generate
      |     sm_TARGET_dout_i(C_S_AXI_DATA_WIDTH-1 downto 32) <= (others => '0');
      | end generate gen_sm_TARGET_dout_i;
      | sm_TARGET_dout_i(32-1 downto 0) <= sm_TARGET_dout;
      | -- 'CONFIG'
      | sm_CONFIG_din     <= sm_CONFIG_din_i(32-1 downto 0);
      | sm_CONFIG_en      <= sm_CONFIG_en_i;
      | gen_sm_CONFIG_dout_i: if (32 < C_S_AXI_DATA_WIDTH) generate
      |     sm_CONFIG_dout_i(C_S_AXI_DATA_WIDTH-1 downto 32) <= (others => '0');
      | end generate gen_sm_CONFIG_dout_i;
      | sm_CONFIG_dout_i(32-1 downto 0) <= sm_CONFIG_dout;
      | -- 'RESET_MODE'
      | sm_RESET_MODE_din     <= sm_RESET_MODE_din_i(32-1 downto 0);
      | sm_RESET_MODE_en      <= sm_RESET_MODE_en_i;
      | gen_sm_RESET_MODE_dout_i: if (32 < C_S_AXI_DATA_WIDTH) generate
      |     sm_RESET_MODE_dout_i(C_S_AXI_DATA_WIDTH-1 downto 32) <= (others => '0');
      | end generate gen_sm_RESET_MODE_dout_i;
      | sm_RESET_MODE_dout_i(32-1 downto 0) <= sm_RESET_MODE_dout;
      | -- 'AGC_OVERRIDE'
      | sm_AGC_OVERRIDE_din     <= sm_AGC_OVERRIDE_din_i(32-1 downto 0);
      | sm_AGC_OVERRIDE_en      <= sm_AGC_OVERRIDE_en_i;
      | gen_sm_AGC_OVERRIDE_dout_i: if (32 < C_S_AXI_DATA_WIDTH) generate
      |     sm_AGC_OVERRIDE_dout_i(C_S_AXI_DATA_WIDTH-1 downto 32) <= (others => '0');
      | end generate gen_sm_AGC_OVERRIDE_dout_i;
      | sm_AGC_OVERRIDE_dout_i(32-1 downto 0) <= sm_AGC_OVERRIDE_dout;
      | -- 'RX_LENGTH'
      | sm_RX_LENGTH_din     <= sm_RX_LENGTH_din_i(32-1 downto 0);
      | sm_RX_LENGTH_en      <= sm_RX_LENGTH_en_i;
      | gen_sm_RX_LENGTH_dout_i: if (32 < C_S_AXI_DATA_WIDTH) generate
      |     sm_RX_LENGTH_dout_i(C_S_AXI_DATA_WIDTH-1 downto 32) <= (others => '0');
      | end generate gen_sm_RX_LENGTH_dout_i;
      | sm_RX_LENGTH_dout_i(32-1 downto 0) <= sm_RX_LENGTH_dout;
      | -- 'TIMING_DCO'
      | sm_TIMING_DCO_din     <= sm_TIMING_DCO_din_i(32-1 downto 0);
      | sm_TIMING_DCO_en      <= sm_TIMING_DCO_en_i;
      | gen_sm_TIMING_DCO_dout_i: if (32 < C_S_AXI_DATA_WIDTH) generate
      |     sm_TIMING_DCO_dout_i(C_S_AXI_DATA_WIDTH-1 downto 32) <= (others => '0');
      | end generate gen_sm_TIMING_DCO_dout_i;
      | sm_TIMING_DCO_dout_i(32-1 downto 0) <= sm_TIMING_DCO_dout;
      | -- 'From FIFO'
      | -- 'To FIFO'
      | -- 'Shared Memory'
      | 
      | ReadWriteSelect: process(memmap_state) is begin
      |     if (memmap_state = READ) then
      |     else
      |     end if;
      | end process ReadWriteSelect;
      | 
      | -----------------------------------------------------------------------------
      | -- address for 'Shared Memory'
      | -----------------------------------------------------------------------------
      | SharedMemory_Addr_ResetN : process(AXI_AClk) is begin
      |     if (AXI_AClk'event and AXI_AClk = '1') then
      |         if (AXI_AResetN = '0') then
      |             memmap_state <= READ;
      |         else
      |             if (S_AXI_AWVALID = '1') then
      |                 -- write operation
      |                 memmap_state <= WRITE;
      |             elsif (S_AXI_ARVALID = '1') then
      |                 -- read operation
      |                 memmap_state <= READ;
      |             end if;
      |         end if;
      |     end if;
      | end process SharedMemory_Addr_ResetN;
      | 
      | -----------------------------------------------------------------------------
      | -- WRITE Command Control
      | -----------------------------------------------------------------------------
      | S_AXI_BID     <= S_AXI_BID_i;
      | S_AXI_BVALID  <= S_AXI_BVALID_i;
      | S_AXI_WREADY  <= S_AXI_WREADY_i;
      | -- No error checking
      | S_AXI_BRESP  <= (others=>'0');
      | 
      | PROC_AWREADY_ACK: process(read_state, write_state, S_AXI_ARVALID, S_AXI_AWVALID) is begin
      |     if (write_state = IDLE and S_AXI_AWVALID = '1' and read_state = IDLE) then
      |         S_AXI_AWREADY <= S_AXI_AWVALID;
      |     else
      |         S_AXI_AWREADY <= '0';
      |     end if;
      | end process PROC_AWREADY_ACK;
      | 
      | Cmd_Decode_Write: process(AXI_AClk) is begin
      |     if (AXI_AClk'event and AXI_AClk = '1') then
      |         if (AXI_AResetN = '0') then
      |             write_addr_valid    <= '0';
      |             write_ready         <= '0';
      |             s_fifo_we           <= '0';
      |             S_AXI_BVALID_i      <= '0';
      |             S_AXI_BID_i         <= (others => '0');
      |             write_bank_addr_i   <= (others => '0');
      |             write_linear_addr_i <= (others => '0');
      |         else
      |             if (write_state = IDLE) then
      |                 if (S_AXI_AWVALID = '1' and read_state = IDLE) then
      |                     -- reflect awid
      |                     S_AXI_BID_i <= S_AXI_AWID;
      | 
      |                     -- latch bank and linear addresses
      |                     write_bank_addr_i   <= S_AXI_AWADDR(C_S_AXI_TOTAL_ADDR_LEN-1 downto C_S_AXI_LINEAR_ADDR_LEN+2);
      |                     write_linear_addr_i <= S_AXI_AWADDR(C_S_AXI_LINEAR_ADDR_LEN+1 downto 2);
      |                     write_addr_valid <= '1';
      |                     s_fifo_we <= '1';
      | 
      |                     -- write state transition
      |                     write_state <= WRITE_DATA;
      |                 end if;
      |             elsif (write_state = WRITE_DATA) then
      |                 write_ready <= '1';
      |                 s_fifo_we <= '0';
      |                 write_addr_valid <= S_AXI_WVALID;
      |                 
      |                 if (S_AXI_WVALID = '1' and write_ready = '1') then
      |                     write_linear_addr_i <= Std_Logic_Vector(unsigned(write_linear_addr_i) + 1);
      |                 end if;
      | 
      |                 if (S_AXI_WLAST = '1' and write_ready = '1') then
      |                     -- start responding through B channel upon the last write data sample
      |                     S_AXI_BVALID_i <= '1';
      |                     -- write data is over
      |                     write_addr_valid <= '0';
      |                     write_ready <= '0';
      |                     -- write state transition
      |                     write_state <= WRITE_RESPONSE;
      |                 end if;
      |             elsif (write_state = WRITE_RESPONSE) then
      | 
      |                 if (S_AXI_BREADY = '1') then
      |                     -- write respond is over
      |                     S_AXI_BVALID_i <= '0';
      |                     S_AXI_BID_i <= (others => '0');
      | 
      |                     -- write state transition
      |                     write_state <= IDLE;
      |                 end if;
      |             end if;
      |         end if;
      |     end if;
      | end process Cmd_Decode_Write;
      | 
      | Write_Linear_Addr_Decode : process(AXI_AClk) is 
      | 
      | begin
      |     if (AXI_AClk'event and AXI_AClk = '1') then
      |         if (AXI_AResetN = '0') then
      |             -- 'To Register'
      |             -- TIMING_RESET din/en
      |             sm_TIMING_RESET_din_i <= (others => '0');
      |             sm_TIMING_RESET_en_i <= '0';
      |             -- RSSI_PWR_CALIB din/en
      |             sm_RSSI_PWR_CALIB_din_i <= (others => '0');
      |             sm_RSSI_PWR_CALIB_en_i <= '0';
      |             -- IIR_COEF_B0 din/en
      |             sm_IIR_COEF_B0_din_i <= (others => '0');
      |             sm_IIR_COEF_B0_en_i <= '0';
      |             -- IIR_COEF_A1 din/en
      |             sm_IIR_COEF_A1_din_i <= (others => '0');
      |             sm_IIR_COEF_A1_en_i <= '0';
      |             -- RESET din/en
      |             sm_RESET_din_i <= (others => '0');
      |             sm_RESET_en_i <= '0';
      |             -- TIMING_AGC din/en
      |             sm_TIMING_AGC_din_i <= (others => '0');
      |             sm_TIMING_AGC_en_i <= '0';
      |             -- TARGET din/en
      |             sm_TARGET_din_i <= (others => '0');
      |             sm_TARGET_en_i <= '0';
      |             -- CONFIG din/en
      |             sm_CONFIG_din_i <= (others => '0');
      |             sm_CONFIG_en_i <= '0';
      |             -- RESET_MODE din/en
      |             sm_RESET_MODE_din_i <= (others => '0');
      |             sm_RESET_MODE_en_i <= '0';
      |             -- AGC_OVERRIDE din/en
      |             sm_AGC_OVERRIDE_din_i <= (others => '0');
      |             sm_AGC_OVERRIDE_en_i <= '0';
      |             -- RX_LENGTH din/en
      |             sm_RX_LENGTH_din_i <= (others => '0');
      |             sm_RX_LENGTH_en_i <= '0';
      |             -- TIMING_DCO din/en
      |             sm_TIMING_DCO_din_i <= (others => '0');
      |             sm_TIMING_DCO_en_i <= '0';
      |             -- 'To FIFO'
      |             -- 'Shared Memory'
      |         else
      |             -- default assignments
      | 
      |             -- 'To Register'
      |             if (unsigned(write_bank_addr_i) = 2) then
      |                 if (unsigned(write_linear_addr_i) = 0) then
      |                     -- TIMING_RESET din/en
      |                     sm_TIMING_RESET_din_i <= S_AXI_WDATA;
      |                     sm_TIMING_RESET_en_i  <= write_addr_valid;
      |                 elsif (unsigned(write_linear_addr_i) = 1) then
      |                     -- RSSI_PWR_CALIB din/en
      |                     sm_RSSI_PWR_CALIB_din_i <= S_AXI_WDATA;
      |                     sm_RSSI_PWR_CALIB_en_i  <= write_addr_valid;
      |                 elsif (unsigned(write_linear_addr_i) = 2) then
      |                     -- IIR_COEF_B0 din/en
      |                     sm_IIR_COEF_B0_din_i <= S_AXI_WDATA;
      |                     sm_IIR_COEF_B0_en_i  <= write_addr_valid;
      |                 elsif (unsigned(write_linear_addr_i) = 3) then
      |                     -- IIR_COEF_A1 din/en
      |                     sm_IIR_COEF_A1_din_i <= S_AXI_WDATA;
      |                     sm_IIR_COEF_A1_en_i  <= write_addr_valid;
      |                 elsif (unsigned(write_linear_addr_i) = 4) then
      |                     -- RESET din/en
      |                     sm_RESET_din_i <= S_AXI_WDATA;
      |                     sm_RESET_en_i  <= write_addr_valid;
      |                 elsif (unsigned(write_linear_addr_i) = 5) then
      |                     -- TIMING_AGC din/en
      |                     sm_TIMING_AGC_din_i <= S_AXI_WDATA;
      |                     sm_TIMING_AGC_en_i  <= write_addr_valid;
      |                 elsif (unsigned(write_linear_addr_i) = 6) then
      |                     -- TARGET din/en
      |                     sm_TARGET_din_i <= S_AXI_WDATA;
      |                     sm_TARGET_en_i  <= write_addr_valid;
      |                 elsif (unsigned(write_linear_addr_i) = 7) then
      |                     -- CONFIG din/en
      |                     sm_CONFIG_din_i <= S_AXI_WDATA;
      |                     sm_CONFIG_en_i  <= write_addr_valid;
      |                 elsif (unsigned(write_linear_addr_i) = 8) then
      |                     -- RESET_MODE din/en
      |                     sm_RESET_MODE_din_i <= S_AXI_WDATA;
      |                     sm_RESET_MODE_en_i  <= write_addr_valid;
      |                 elsif (unsigned(write_linear_addr_i) = 9) then
      |                     -- AGC_OVERRIDE din/en
      |                     sm_AGC_OVERRIDE_din_i <= S_AXI_WDATA;
      |                     sm_AGC_OVERRIDE_en_i  <= write_addr_valid;
      |                 elsif (unsigned(write_linear_addr_i) = 10) then
      |                     -- RX_LENGTH din/en
      |                     sm_RX_LENGTH_din_i <= S_AXI_WDATA;
      |                     sm_RX_LENGTH_en_i  <= write_addr_valid;
      |                 elsif (unsigned(write_linear_addr_i) = 11) then
      |                     -- TIMING_DCO din/en
      |                     sm_TIMING_DCO_din_i <= S_AXI_WDATA;
      |                     sm_TIMING_DCO_en_i  <= write_addr_valid;
      |                 end if;
      |             end if;        
      |         
      |         
      |         end if;
      |     end if;
      | end process Write_Linear_Addr_Decode;
      |  
      | -----------------------------------------------------------------------------
      | -- READ Control
      | -----------------------------------------------------------------------------
      | 
      | S_AXI_RDATA  <= S_AXI_RDATA_i;
      | S_AXI_RVALID  <= S_AXI_RVALID_i;
      | S_AXI_RLAST   <= S_AXI_RLAST_i;
      | S_AXI_RID     <= S_AXI_RID_i;
      | -- TODO: no error checking
      | S_AXI_RRESP <= (others=>'0');
      | 
      | PROC_ARREADY_ACK: process(read_state, S_AXI_ARVALID, write_state, S_AXI_AWVALID) is begin
      |     -- Note: WRITE has higher priority than READ
      |     if (read_state = IDLE and S_AXI_ARVALID = '1' and write_state = IDLE and S_AXI_AWVALID /= '1') then
      |         S_AXI_ARREADY <= S_AXI_ARVALID;
      |     else
      |         S_AXI_ARREADY <= '0';
      |     end if;
      | end process PROC_ARREADY_ACK;
      | 
      | S_AXI_WREADY_i <= write_ready;
      | 
      | Process_Sideband: process(write_state, read_state) is begin
      |     if (read_state = READ_PREP) then
      |         s_shram_en <= '1';
      |     elsif (read_state = READ_DATA) then
      |         s_shram_en <= S_AXI_RREADY;
      |     elsif (write_state = WRITE_DATA) then
      |         s_shram_en <= S_AXI_WVALID;
      |     else
      |         s_shram_en <= '0';
      |     end if;
      | end process Process_Sideband;
      | 
      | Cmd_Decode_Read: process(AXI_AClk) is begin
      |     if (AXI_AClk'event and AXI_AClk = '1') then
      |         if (AXI_AResetN = '0') then
      |             S_AXI_RVALID_i <= '0';
      |             read_bank_addr_i    <= (others => '0');
      |             read_linear_addr_i  <= (others => '0');
      |             S_AXI_ARLEN_i       <= (others => '0');
      |             S_AXI_RLAST_i       <= '0';
      |             S_AXI_RID_i         <= (others => '0');
      |             read_state          <= IDLE;
      |             read_prep_counter   <= (others => '0');
      |             read_addr_counter   <= (others => '0');
      |             read_data_counter   <= (others => '0');
      |         else
      |             -- default assignments
      |             s_fifo_re <= '0';
      | 
      |             if (read_state = IDLE) then
      |                 -- Note WRITE has higher priority than READ
      |                 if (S_AXI_ARVALID = '1' and write_state = IDLE and S_AXI_AWVALID /= '1') then
      |                     -- extract bank and linear addresses
      |                     read_bank_addr_i    <= S_AXI_ARADDR(C_S_AXI_TOTAL_ADDR_LEN-1 downto C_S_AXI_LINEAR_ADDR_LEN+2);
      |                     read_linear_addr_i  <= S_AXI_ARADDR(C_S_AXI_LINEAR_ADDR_LEN+1 downto 2);
      |                     s_fifo_re <= '1';
      | 
      |                     -- reflect arid
      |                     S_AXI_RID_i <= S_AXI_ARID;
      | 
      |                     -- load read liner address and data counter
      |                     read_addr_counter <= S_AXI_ARLEN;
      |                     read_data_counter <= S_AXI_ARLEN;
      | 
      |                     -- load read preparation counter
      |                     read_prep_counter <= C_READ_PREP_DELAY;
      |                     -- read state transition
      |                     read_state <= READ_PREP;
      |                 end if;
      |             elsif (read_state = READ_PREP) then
      |                 if (unsigned(read_prep_counter) = 0) then
      |                     if (unsigned(read_data_counter) = 0) then
      |                         -- tag the last data generated by the slave
      |                         S_AXI_RLAST_i <= '1';
      |                     end if;
      |                     -- valid data appears
      |                     S_AXI_RVALID_i <= '1';
      |                     -- read state transition
      |                     read_state <= READ_DATA;
      |                 else
      |                     -- decrease read preparation counter
      |                     read_prep_counter <= Std_Logic_Vector(unsigned(read_prep_counter) - 1);
      |                 end if;
      | 
      |                 if (unsigned(read_prep_counter) /= 3 and unsigned(read_addr_counter) /= 0) then
      |                     -- decrease address counter
      |                     read_addr_counter <= Std_Logic_Vector(unsigned(read_addr_counter) - 1);
      |                     -- increase linear address (no band crossing)
      |                     read_linear_addr_i <= Std_Logic_Vector(unsigned(read_linear_addr_i) + 1);
      |                 end if;
      |             elsif (read_state = READ_DATA) then
      |                 if (S_AXI_RREADY = '1') then
      |                     if (unsigned(read_data_counter) = 1) then
      |                         -- tag the last data generated by the slave
      |                         S_AXI_RLAST_i <= '1';
      |                     end if;
      | 
      |                     if (unsigned(read_data_counter) = 0) then
      |                         -- arid
      |                         S_AXI_RID_i <= (others => '0');
      |                         -- rlast
      |                         S_AXI_RLAST_i <= '0';
      |                         -- no more valid data
      |                         S_AXI_RVALID_i <= '0';
      |                         -- read state transition
      |                         read_state <= IDLE;
      |                     else
      |                         -- decrease read preparation counter
      |                         read_data_counter <= Std_Logic_Vector(unsigned(read_data_counter) - 1);
      | 
      |                         if (unsigned(read_addr_counter) /= 0) then
      |                             -- decrease address counter
      |                             read_addr_counter <= Std_Logic_Vector(unsigned(read_addr_counter) - 1);
      |                             -- increase linear address (no band crossing)
      |                             read_linear_addr_i <= Std_Logic_Vector(unsigned(read_linear_addr_i) + 1);
      |                         end if;
      |                     end if;
      |                 end if;
      |             end if;
      | 
      |         end if;
      |     end if;
      | end process Cmd_Decode_Read;
      | 
      | Read_Linear_Addr_Decode : process(AXI_AClk) is begin
      |     if (AXI_AClk'event and AXI_AClk = '1') then
      |         if (AXI_AResetN = '0') then
      |             reg_bank_out_i   <= (others => '0');
      |             fifo_bank_out_i  <= (others => '0');
      |             shmem_bank_out_i <= (others => '0');
      |             S_AXI_RDATA_i    <= (others => '0');
      |         else
      |             if (unsigned(read_bank_addr_i) = 2) then
      |                 -- 'From Register'
      |                 -- 'To Register' (with register readback)
      |                 if (unsigned(read_linear_addr_i) = 0) then
      |                     -- 'TIMING_RESET' dout
      |                     reg_bank_out_i <= sm_TIMING_RESET_dout_i;
      |                 elsif (unsigned(read_linear_addr_i) = 1) then
      |                     -- 'RSSI_PWR_CALIB' dout
      |                     reg_bank_out_i <= sm_RSSI_PWR_CALIB_dout_i;
      |                 elsif (unsigned(read_linear_addr_i) = 2) then
      |                     -- 'IIR_COEF_B0' dout
      |                     reg_bank_out_i <= sm_IIR_COEF_B0_dout_i;
      |                 elsif (unsigned(read_linear_addr_i) = 3) then
      |                     -- 'IIR_COEF_A1' dout
      |                     reg_bank_out_i <= sm_IIR_COEF_A1_dout_i;
      |                 elsif (unsigned(read_linear_addr_i) = 4) then
      |                     -- 'RESET' dout
      |                     reg_bank_out_i <= sm_RESET_dout_i;
      |                 elsif (unsigned(read_linear_addr_i) = 5) then
      |                     -- 'TIMING_AGC' dout
      |                     reg_bank_out_i <= sm_TIMING_AGC_dout_i;
      |                 elsif (unsigned(read_linear_addr_i) = 6) then
      |                     -- 'TARGET' dout
      |                     reg_bank_out_i <= sm_TARGET_dout_i;
      |                 elsif (unsigned(read_linear_addr_i) = 7) then
      |                     -- 'CONFIG' dout
      |                     reg_bank_out_i <= sm_CONFIG_dout_i;
      |                 elsif (unsigned(read_linear_addr_i) = 8) then
      |                     -- 'RESET_MODE' dout
      |                     reg_bank_out_i <= sm_RESET_MODE_dout_i;
      |                 elsif (unsigned(read_linear_addr_i) = 9) then
      |                     -- 'AGC_OVERRIDE' dout
      |                     reg_bank_out_i <= sm_AGC_OVERRIDE_dout_i;
      |                 elsif (unsigned(read_linear_addr_i) = 10) then
      |                     -- 'RX_LENGTH' dout
      |                     reg_bank_out_i <= sm_RX_LENGTH_dout_i;
      |                 elsif (unsigned(read_linear_addr_i) = 11) then
      |                     -- 'TIMING_DCO' dout
      |                     reg_bank_out_i <= sm_TIMING_DCO_dout_i;
      |                 end if;
      | 
      |                 S_AXI_RDATA_i <= reg_bank_out_i;
      |             elsif (unsigned(read_bank_addr_i) = 1) then
      |                 -- 'From FIFO'
      |                 -- 'To FIFO'
      | 
      |                 S_AXI_RDATA_i <= fifo_bank_out_i;
      |             elsif (unsigned(read_bank_addr_i) = 0 and s_shram_en = '1') then
      |                 -- 'Shared Memory'
      | 
      |                 S_AXI_RDATA_i <= shmem_bank_out_i;
      |             end if;
      |         end if;
      |     end if;
      | end process Read_Linear_Addr_Decode;
      | 
      | end architecture IMP;
      settings: infoedit=For use with EDK Processor block.
  wires:
  memmap/13 -> To Register/2
  memmap/12 -> To Register/1
  memmap/35 -> To Register11/2
  memmap/34 -> To Register11/1
  memmap/23 -> To Register5/2
  memmap/22 -> To Register5/1
  memmap/25 -> To Register6/2
  memmap/24 -> To Register6/1
  memmap/33 -> To Register10/2
  memmap/32 -> To Register10/1
  memmap/15 -> To Register1/2
  memmap/14 -> To Register1/1
  memmap/21 -> To Register4/2
  memmap/20 -> To Register4/1
  memmap/29 -> To Register8/2
  memmap/28 -> To Register8/1
  memmap/17 -> To Register2/2
  memmap/16 -> To Register2/1
  memmap/19 -> To Register3/2
  memmap/18 -> To Register3/1
  memmap/27 -> To Register7/2
  memmap/26 -> To Register7/1
  memmap/31 -> To Register9/2
  memmap/30 -> To Register9/1
  memmap/11 -> S_AXI_WREADY/1
  memmap/10 -> S_AXI_RVALID/1
  memmap/9 -> S_AXI_RRESP/1
  memmap/8 -> S_AXI_RLAST/1
  memmap/7 -> S_AXI_RID/1
  memmap/6 -> S_AXI_RDATA/1
  memmap/5 -> S_AXI_BVALID/1
  memmap/4 -> S_AXI_BRESP/1
  memmap/3 -> S_AXI_BID/1
  memmap/2 -> S_AXI_AWREADY/1
  memmap/1 -> S_AXI_ARREADY/1
  S_AXI_WVALID/1 -> memmap/25
  S_AXI_WSTRB/1 -> memmap/24
  S_AXI_WLAST/1 -> memmap/23
  S_AXI_WDATA/1 -> memmap/22
  S_AXI_RREADY/1 -> memmap/21
  S_AXI_BREADY/1 -> memmap/20
  S_AXI_AWVALID/1 -> memmap/19
  S_AXI_AWSIZE/1 -> memmap/18
  S_AXI_AWPROT/1 -> memmap/17
  S_AXI_AWLOCK/1 -> memmap/16
  S_AXI_AWLEN/1 -> memmap/15
  S_AXI_AWID/1 -> memmap/14
  S_AXI_AWCACHE/1 -> memmap/13
  S_AXI_AWBURST/1 -> memmap/12
  S_AXI_AWADDR/1 -> memmap/11
  S_AXI_ARVALID/1 -> memmap/10
  S_AXI_ARSIZE/1 -> memmap/9
  S_AXI_ARPROT/1 -> memmap/8
  S_AXI_ARLOCK/1 -> memmap/7
  S_AXI_ARLEN/1 -> memmap/6
  S_AXI_ARID/1 -> memmap/5
  S_AXI_ARCACHE/1 -> memmap/4
  S_AXI_ARBURST/1 -> memmap/3
  S_AXI_ARADDR/1 -> memmap/2
  AXI_ARESETN/1 -> memmap/1
  To Register/1 -> memmap/26
  To Register11/1 -> memmap/37
  To Register5/1 -> memmap/31
  To Register6/1 -> memmap/32
  To Register10/1 -> memmap/36
  To Register1/1 -> memmap/27
  To Register4/1 -> memmap/30
  To Register8/1 -> memmap/34
  To Register2/1 -> memmap/28
  To Register3/1 -> memmap/29
  To Register7/1 -> memmap/33
  To Register9/1 -> memmap/35
  S_AXI_WREADY/1 -> Terminator10/1
  S_AXI_RVALID/1 -> Terminator9/1
  S_AXI_RRESP/1 -> Terminator8/1
  S_AXI_RLAST/1 -> Terminator7/1
  S_AXI_RID/1 -> Terminator6/1
  S_AXI_RDATA/1 -> Terminator5/1
  S_AXI_BVALID/1 -> Terminator4/1
  S_AXI_BRESP/1 -> Terminator3/1
  S_AXI_BID/1 -> Terminator2/1
  S_AXI_AWREADY/1 -> Terminator1/1
  S_AXI_ARREADY/1 -> Terminator/1
  Constant24/1 -> S_AXI_WVALID/1
  Constant23/1 -> S_AXI_WSTRB/1
  Constant22/1 -> S_AXI_WLAST/1
  Constant21/1 -> S_AXI_WDATA/1
  Constant20/1 -> S_AXI_RREADY/1
  Constant19/1 -> S_AXI_BREADY/1
  Constant18/1 -> S_AXI_AWVALID/1
  Constant17/1 -> S_AXI_AWSIZE/1
  Constant16/1 -> S_AXI_AWPROT/1
  Constant15/1 -> S_AXI_AWLOCK/1
  Constant14/1 -> S_AXI_AWLEN/1
  Constant13/1 -> S_AXI_AWID/1
  Constant12/1 -> S_AXI_AWCACHE/1
  Constant11/1 -> S_AXI_AWBURST/1
  Constant10/1 -> S_AXI_AWADDR/1
  Constant9/1 -> S_AXI_ARVALID/1
  Constant8/1 -> S_AXI_ARSIZE/1
  Constant7/1 -> S_AXI_ARPROT/1
  Constant6/1 -> S_AXI_ARLOCK/1
  Constant5/1 -> S_AXI_ARLEN/1
  Constant4/1 -> S_AXI_ARID/1
  Constant3/1 -> S_AXI_ARCACHE/1
  Constant2/1 -> S_AXI_ARBURST/1
  Constant1/1 -> S_AXI_ARADDR/1
  Constant/1 -> AXI_ARESETN/1
